simulink model "fig2_8_pio"  (R2026a)
settings: Solver=ode15s  StopTime=7  MaxStep=0.005  RelTol=1e-6  AbsTol=1e-8
values from neighbouring files (symbols this model uses):
  denGac = conv(conv([1 2*0.212*0.088 0.088^2],[1 3.75]),[1 -1.44])    [reproduce_fig2_8_time_domain.m]
  denGc = conv(conv([1 2*0.442*22.85 22.85^2],[1 0]),[1 1.16])    [reproduce_fig2_8_time_domain.m]
  numGac = -10.524 * conv(conv([1 1.562],[1 0.038]),[1 0])    [reproduce_fig2_8_time_domain.m]
  numGc = 5.21 * conv(conv([1 -57.36],[1 4.26]),[1 0.55])    [reproduce_fig2_8_time_domain.m]
  qco = 1.1    [reproduce_fig2_8_time_domain.m]
  R = 60    [reproduce_fig2_8_time_domain.m]
  w = omegas(j)    [reproduce_fig2_8_time_domain.m]
settings Model: Creator=t0900  LastModifiedBy=t0900

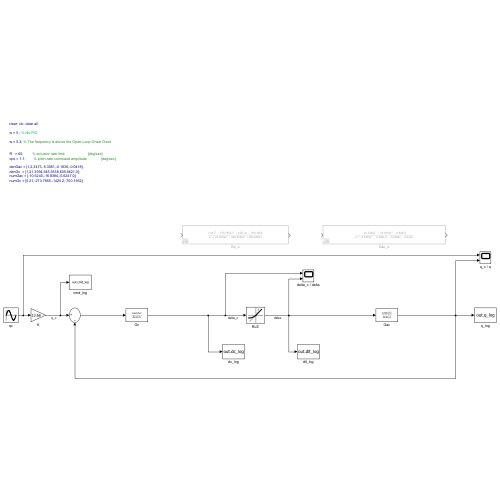
[thumbnail: Simulink's stored preview of the top-level diagram]
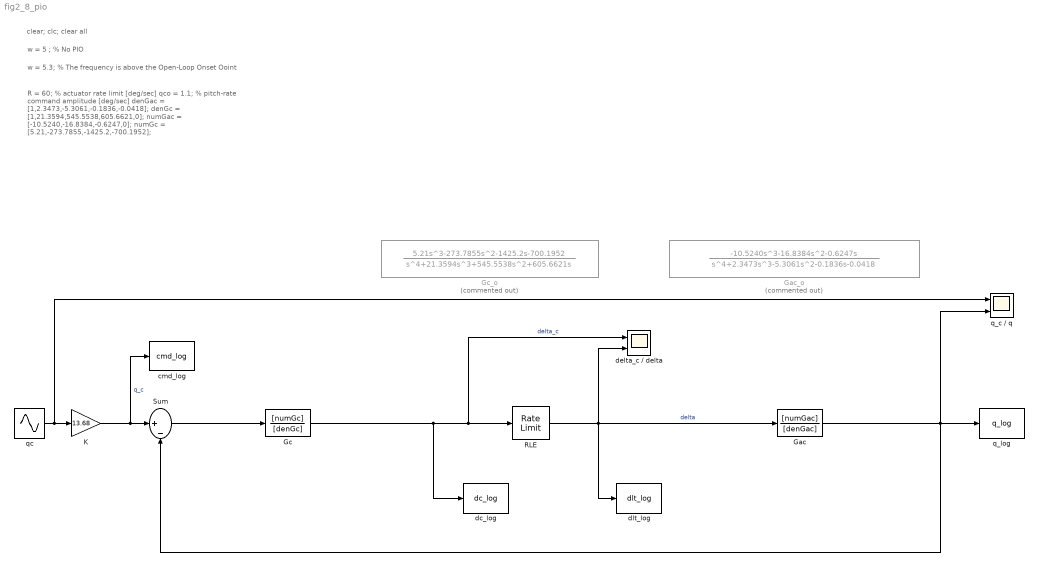
== system fig2_8_pio ==
  note: R   = 60;         % actuator rate limit                       [deg/sec]
      | qco = 1.1;        % pitch-rate command amplitude              [deg/sec]
      |
      | denGac = [1,2.3473,-5.3061,-0.1836,-0.0418];
      | denGc  = [1,21.3594,545.5538,605.6621,0];
      | numGac = [-10.5240,-16.8384,-0.6247,0];
      | numGc = [5.21,-273.7855,-1425.2,-700.1952];
  note: clear; clc; clear all
  note: w = 5.3; % The frequency is above the Open-Loop Onset Ooint
  note: w = 5 ; % No PIO
  Gac : TransferFcn  Numerator=[numGac]  Denominator=[denGac]
  Gac_o : TransferFcn  Commented=on  Numerator=[-10.5240,-16.8384,-0.6247,0]  Denominator=[1,2.3473,-5.3061,-0.1836,-0.0418]
  Gc : TransferFcn  Numerator=[numGc]  Denominator=[denGc]
  Gc_o : TransferFcn  Commented=on  Numerator=[5.21,-273.7855,-1425.2,-700.1952]  Denominator=[1,21.3594,545.5538,605.6621,0]
  K : Gain  Gain=13.68
  RLE : RateLimiter  RisingSlewLimit=R  FallingSlewLimit=-R  SampleTimeMode=inherited
  Sum : Sum  Inputs=|+-
  cmd_log : ToWorkspace  VariableName=cmd_log  SaveFormat=Timeseries  SampleTime=-1
  dc_log : ToWorkspace  VariableName=dc_log  SaveFormat=Timeseries  SampleTime=-1
  delta_c / delta : Scope  NumInputPorts=2
      settings: ActiveDisplayYMinimum=-16.68841288079388  ActiveDisplayYMaximum=16.709980059570565
  dlt_log : ToWorkspace  VariableName=dlt_log  SaveFormat=Timeseries  SampleTime=-1
  q_c / q : Scope  NumInputPorts=2
      settings: ActiveDisplayYMinimum=-28.099384588496545  ActiveDisplayYMaximum=27.647903593911231
  q_log : ToWorkspace  VariableName=q_log  SaveFormat=Timeseries  SampleTime=-1
  qc : Sin  Amplitude=qco  Frequency=w  SampleTime=0
  wires:
  qc/1 -> q_c / q/1, K/1
  K/1 -> Sum/1, cmd_log/1  "q_c"
  Sum/1 -> Gc/1
  Gc/1 -> delta_c / delta/1, RLE/1, dc_log/1  "delta_c"
  RLE/1 -> Gac/1, delta_c / delta/2, dlt_log/1  "delta"
  Gac/1 -> q_log/1, Sum/2, q_c / q/2
